simulink model "sf_bouncing_2018a"  (R2018a)
settings: Solver=VariableStepAuto  StartTime=0.0  StopTime=10.0  RelTol=1e-3
settings Model: Creator=bzhan  LastModifiedBy=bzhan
settings DataIOCC: ReturnWorkspaceOutputs=on
settings SFSimCC: SimUseLocalCustomCode=on
settings RTWCC: RTWUseLocalCustomCode=on

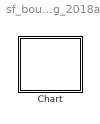
== system sf_bouncing_2018a ==
  Chart : Stateflow chart  TreatAsAtomicUnit=on

== stateflow chart sf_bouncing_2018a/Chart ==
  settings: updateMethod=CONTINUOUS
  state A
    du: x_dot=v; v_dot=a;
  (default) -> A : {x=5;v=0;a=-9.8;}
  A -> A : [x<=0&&v<=0]{v=-0.9*v;}
  data: v local; a local; x local
  data v settings: updateMethod=SF_CONTINUOUS_TIME_DATA
  data a settings: updateMethod=SF_CONTINUOUS_TIME_DATA
  data x settings: updateMethod=SF_CONTINUOUS_TIME_DATA
